simulink model "hw3_simulink"  (R2021b)
settings: Solver=VariableStepAuto  StartTime=0.0  StopTime=10.0  RelTol=1e-3
settings Model: Creator=Parsa_The_Conqeuror  LastModifiedBy=Parsa_The_Conqeuror

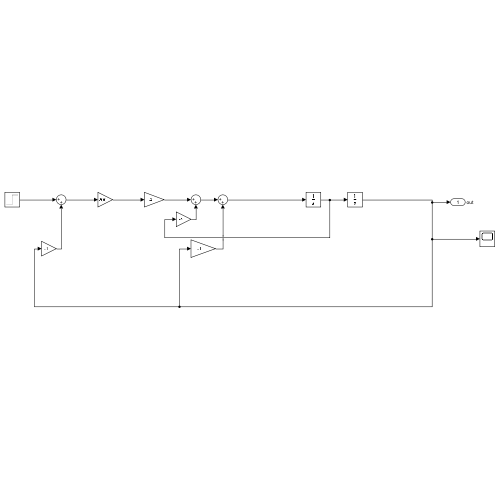
[thumbnail: Simulink's stored preview of the top-level diagram]
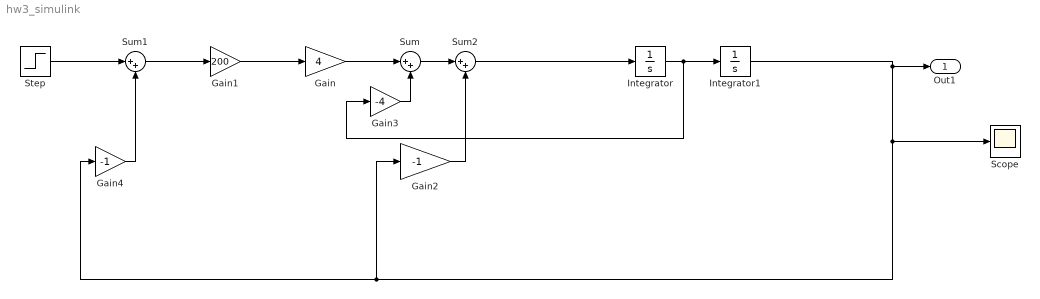
== system hw3_simulink ==
  Gain : Gain  Gain=4
  Gain1 : Gain  Gain=200
  Gain2 : Gain  Gain=-1
  Gain3 : Gain  Gain=-4
  Gain4 : Gain  Gain=-1
  Integrator : Integrator
  Integrator1 : Integrator
  Scope : Scope
  Step : Step  Time=0  SampleTime=0
  Sum : Sum  Inputs=|++
  Sum1 : Sum  Inputs=|++
  Sum2 : Sum  Inputs=|++
  Out1 : Outport  SignalName=out
  wires:
  Gain/1 -> Sum/1
  Gain1/1 -> Gain/1
  Integrator/1 -> Gain3/1, Integrator1/1
  Step/1 -> Sum1/1
  Gain3/1 -> Sum/2
  Sum/1 -> Sum2/1
  Integrator1/1 -> Out1/1, Scope/1, Gain4/1, Gain2/1
  Gain2/1 -> Sum2/2
  Sum2/1 -> Integrator/1
  Gain4/1 -> Sum1/2
  Sum1/1 -> Gain1/1
